simulink model "AnalizaSymulacyjna_z_opoznieniem"  (R2022b)
settings: Solver=VariableStepAuto  StartTime=0.0  StopTime=20  RelTol=1e-3
libraries: slpidlib x3
settings Model: Creator=hpiet  LastModifiedBy=hpiet

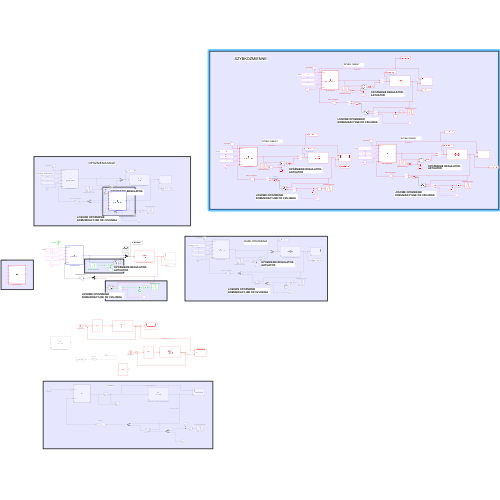
[thumbnail: Simulink's stored preview of the top-level diagram]
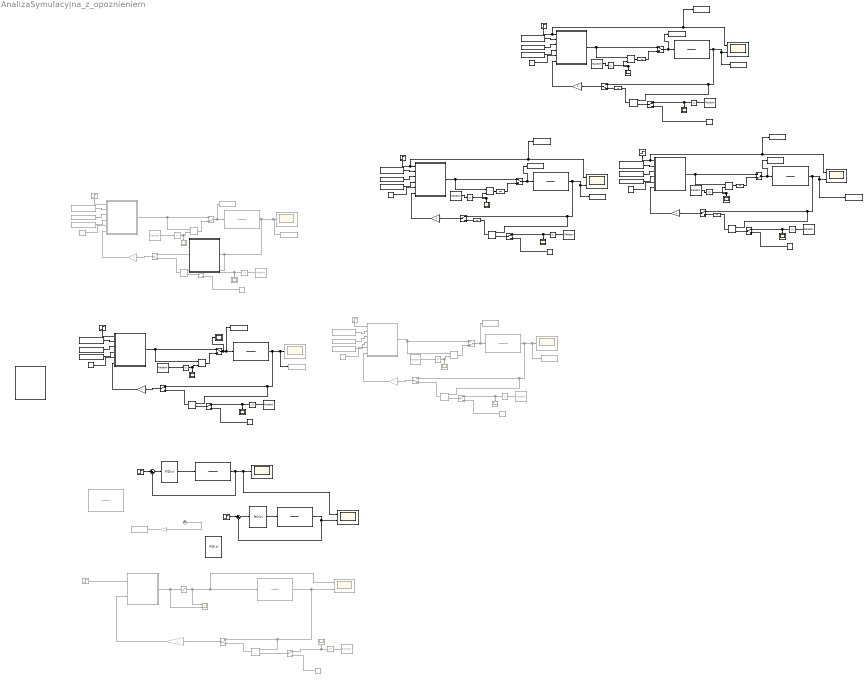
== system AnalizaSymulacyjna_z_opoznieniem ==
  note: SZYBKOZMIENNE
  note: SZYBKI OBIEKT
  note: OPOZNIENIA MALE
  note: WINDUP
  note: ORYGIAL
  note: DUZE OPOZNIENIA
  note: 23.33449541284404
  note: OPÓŹNIENIE REGULATOR-AKTUATOR
  note: LOSOWE OPÓŹNIENIE KOMUNIKACYJNE OD CZUJNIKA
  note: Z SATURACJA
  note: LOSOWE OPÓŹNIENIE KOMUNIKACYJNE OD CZUJNIKA
  note: OPÓŹNIENIE REGULATOR-AKTUATOR
  note: 23.33449541284404
  note: LOSOWE OPÓŹNIENIE KOMUNIKACYJNE OD CZUJNIKA
  note: OPÓŹNIENIE REGULATOR-AKTUATOR
  note: 23.33449541284404
  note: LOSOWE OPÓŹNIENIE KOMUNIKACYJNE OD CZUJNIKA
  note: 23.33449541284404
  note: OPÓŹNIENIE REGULATOR-AKTUATOR
  note: SZYBKI OBIEKT
  note: 23.33449541284404
  note: OPÓŹNIENIE REGULATOR-AKTUATOR
  note: LOSOWE OPÓŹNIENIE KOMUNIKACYJNE OD CZUJNIKA
  note: SZYBKI OBIEKT
  note: 23.33449541284404
  note: OPÓŹNIENIE REGULATOR-AKTUATOR
  note: LOSOWE OPÓŹNIENIE KOMUNIKACYJNE OD CZUJNIKA
  Abs{1,3,8..13} (8 alike) : Abs  SaturateOnIntegerOverflow=off
  Abs{2,4..7} (5 alike) : Abs  Commented=on  SaturateOnIntegerOverflow=off
  CZUJNIK1 : Gain  Commented=on
  Constant1 : Constant  Commented=on  Value=0.1
  Constant{6..7,10,12} (4 alike) : Constant  Value=0
  Constant{8..9,11,13} (4 alike) : Constant  Value=2
  Constant2 : Constant  Commented=on  Value=3.27
  Constant3 : Constant  Commented=on  Value=2
  Constant4 : Constant  Commented=on  Value=3.27
  Constant5 : Constant  Commented=on  Value=2
  Correction : Gain  Commented=on  Gain=0.1
  Discrete Transfer Fcn1 : DiscreteTransferFcn  Numerator=[0.001667]  Denominator=[1 -1]
  Discrete Transfer Fcn{5..8,10..11} (6 alike) : DiscreteTransferFcn  Denominator=[1]  SampleTime=0.02
  Discrete Transfer Fcn{2..4,9} (4 alike) : DiscreteTransferFcn  Numerator=[0.129]  Denominator=[1 -0.9355]  SampleTime=0.02
  "Example slow-changing plant " : TransferFcn  Commented=on  Numerator=[50]  Denominator=[300 1]
  IMITACJA CZUJNIKA{,3..5} (4 alike) : Gain
  IMITACJA CZUJNIKA1 : Gain  Commented=on
  IMITACJA CZUJNIKA2 : Gain  Commented=on
  KI : Constant  Value=1.2
  KI1 : Constant  Commented=on  Value=1.2
  KI2 : Constant  Commented=on  Value=1.2
  KI3 : Constant  Value=0.3
  KI4 : Constant  Value=0.3
  KI5 : Constant  Value=0.3
  KP : Constant  Value=23.3345
  KP1 : Constant  Commented=on  Value=23.33449541284404
  KP2 : Constant  Commented=on  Value=23.33449541284404
  KP3 : Constant  Value=0.08
  KP4 : Constant  Value=0.08
  KP5 : Constant  Value=0.08
  LOSOWE OPÓŹNIENIE1 : RandomNumber  Commented=on  Mean=0.1  Variance=0.0001  SampleTime=0.1
  MATLAB Function1 : MATLAB Function  Commented=on  TreatAsAtomicUnit=on
  Manual Switch{1,4,6..7,9} (5 alike) : ManualSwitch  Commented=on  CurrentSetting=0
  Manual Switch{3,10..16,19..20} (10 alike) : ManualSwitch
  Manual Switch17 : ManualSwitch  CurrentSetting=0
  Manual Switch18 : ManualSwitch  CurrentSetting=0
  Manual Switch2 : ManualSwitch  Commented=on
  Manual Switch5 : ManualSwitch  Commented=on
  Manual Switch8 : ManualSwitch  Commented=on
  PID CONTROLLER : MATLAB Function  TreatAsAtomicUnit=on
  PID CONTROLLER1 : MATLAB Function  Commented=on  TreatAsAtomicUnit=on  SystemSampleTime=0.5
  PID CONTROLLER2 : MATLAB Function  TreatAsAtomicUnit=on  SystemSampleTime=0.02
  PID CONTROLLER3 : MATLAB Function  TreatAsAtomicUnit=on  SystemSampleTime=0.5
  PID CONTROLLER4 : MATLAB Function  TreatAsAtomicUnit=on  SystemSampleTime=0.5
  PID CONTROLLER5 : MATLAB Function  Commented=on  TreatAsAtomicUnit=on  SystemSampleTime=0.5
  PID CONTROLLER6 : MATLAB Function  TreatAsAtomicUnit=on  SystemSampleTime=0.02
  PID CONTROLLER7 : MATLAB Function  TreatAsAtomicUnit=on  SystemSampleTime=0.02
  PID Controller : slpidlib/PID Controller  Controller=PID  Form=Parallel  TimeDomain=Discrete-time  UseExternalTs=off  SampleTime=-1  IntegratorMethod=Forward Euler  FilterMethod=Forward Euler  ControllerParametersSource=internal  P=16.762157558433  I=0.863667240387185  UseKiTs=off  D=11.7329946521911  N=1.01565558025853  UseFilter=on  TunerSelectOption=Transfer Function Based (PID Tuner App)  InitialConditionSource=internal  InitialConditionForIntegrator=0  InitialConditionForFilter=0  DifferentiatorICPrevScaledInput=0  ExternalReset=none  TrackingMode=off  Kt=1  LimitOutput=off  SatLimitsSource=internal  UpperSaturationLimit=inf  LowerSaturationLimit=-inf  LinearizeAsGain=on  AntiWindupMode=none  Kb=1  LimitIntegrator=off  UpperIntegratorSaturationLimit=inf  LowerIntegratorSaturationLimit=-inf  POutMin=[]  POutMax=[]  IOutMin=[]  IOutMax=[]  DOutMin=[]  DOutMax=[]  NOutMin=[]  NOutMax=[]  SumOutMin=[]  SumOutMax=[]  SaturationOutMin=[]  SaturationOutMax=[]  PParamMin=[]  PParamMax=[]  IParamMin=[]  IParamMax=[]  DParamMin=[]  DParamMax=[]  NParamMin=[]  NParamMax=[]  KbParamMin=[]  KbParamMax=[]  KtParamMin=[]  KtParamMax=[]  KbOutMin=[]  KbOutMax=[]  KtOutMin=[]  KtOutMax=[]  IntegratorOutMin=[]  IntegratorOutMax=[]  FilterOutMin=[]  FilterOutMax=[]  SumI1OutMin=[]  SumI1OutMax=[]  SumI2OutMin=[]  SumI2OutMax=[]  SumI3OutMin=[]  SumI3OutMax=[]  SumI4OutMin=[]  SumI4OutMax=[]  SumDOutMin=[]  SumDOutMax=[]  DifferentiatorOutMin=[]  DifferentiatorOutMax=[]  FilterDiffOutCoefMin=[]  FilterDiffOutCoefMax=[]  ReciprocalOutMin=[]  ReciprocalOutMax=[]  SumDenOutMin=[]  SumDenOutMax=[]  SumNumOutMin=[]  SumNumOutMax=[]  DivideOutMin=[]  DivideOutMax=[]  UdiffTsProdOutMin=[]  UdiffTsProdOutMax=[]  NTsProdOutMin=[]  NTsProdOutMax=[]  UintegralTsProdOutMin=[]  UintegralTsProdOutMax=[]  UngainTsProdOutMin=[]  UngainTsProdOutMax=[]  ClampingZeroOutDataTypeStr=Inherit: Inherit via back propagation  ClampingZeroOutMin=[]  ClampingZeroOutMax=[]  FilterDenConstantOutDataTypeStr=Inherit: Inherit via back propagation  FilterDenConstantOutMin=[]  FilterDenConstantOutMax=[]  PCopyOutDataTypeStr=Inherit: Inherit via back propagation  PCopyOutMin=[]  PCopyOutMax=[]  NCopyOutDataTypeStr=Inherit: Inherit via back propagation  NCopyOutMin=[]  NCopyOutMax=[]  IntegratorContinuousStateAttributes=''  IntegratorStateMustResolveToSignalObject=off  IntegratorRTWStateStorageClass=Auto  FilterContinuousStateAttributes=''  FilterStateMustResolveToSignalObject=off  FilterRTWStateStorageClass=Auto  ParallelPVariant=InternalParameters  IdealPVariant=Disabled  IVariant=InternalParameters  DVariant=InternalParameters  IntegratorVariant=Discrete  SatVariant=Disabled  AWVariant=Passthrough  PCopyVariant=Disabled  TRVariant=Disabled  FdbkBlocksVariant=Forward  IdealPFdbkVariant=Disabled  SatFdbkVariant=Disabled  DerivativeFilterVariant=ForwardEulerFilter  NVariant=InternalParameters  NCopyVariant=Disabled  FilterICVariant=InternalICsFilter  IntegratorICVariant=InternalICs  ExternalResetVariant=Disabled  TRSumVariant=Passthrough  SumFdbkVariant=Disabled  SumVariant=Sum_PID  TsampFilterVariant=InternalTs  TsampNgainVariant=Passthrough  TsampIntegralVariant=Passthrough  ExternalSaturationOutDataTypeStr=Inherit: Same as second input
  PID Controller1 : slpidlib/PID Controller  Controller=PID  Form=Parallel  TimeDomain=Discrete-time  UseExternalTs=off  SampleTime=-1  IntegratorMethod=Forward Euler  FilterMethod=Forward Euler  ControllerParametersSource=internal  P=16.762157558433  I=0.863667240387185  UseKiTs=off  D=11.7329946521911  N=1.01565558025853  UseFilter=on  TunerSelectOption=Transfer Function Based (PID Tuner App)  InitialConditionSource=internal  InitialConditionForIntegrator=0  InitialConditionForFilter=0  DifferentiatorICPrevScaledInput=0  ExternalReset=none  TrackingMode=off  Kt=1  LimitOutput=off  SatLimitsSource=internal  UpperSaturationLimit=inf  LowerSaturationLimit=-inf  LinearizeAsGain=on  AntiWindupMode=none  Kb=1  LimitIntegrator=off  UpperIntegratorSaturationLimit=inf  LowerIntegratorSaturationLimit=-inf  POutMin=[]  POutMax=[]  IOutMin=[]  IOutMax=[]  DOutMin=[]  DOutMax=[]  NOutMin=[]  NOutMax=[]  SumOutMin=[]  SumOutMax=[]  SaturationOutMin=[]  SaturationOutMax=[]  PParamMin=[]  PParamMax=[]  IParamMin=[]  IParamMax=[]  DParamMin=[]  DParamMax=[]  NParamMin=[]  NParamMax=[]  KbParamMin=[]  KbParamMax=[]  KtParamMin=[]  KtParamMax=[]  KbOutMin=[]  KbOutMax=[]  KtOutMin=[]  KtOutMax=[]  IntegratorOutMin=[]  IntegratorOutMax=[]  FilterOutMin=[]  FilterOutMax=[]  SumI1OutMin=[]  SumI1OutMax=[]  SumI2OutMin=[]  SumI2OutMax=[]  SumI3OutMin=[]  SumI3OutMax=[]  SumI4OutMin=[]  SumI4OutMax=[]  SumDOutMin=[]  SumDOutMax=[]  DifferentiatorOutMin=[]  DifferentiatorOutMax=[]  FilterDiffOutCoefMin=[]  FilterDiffOutCoefMax=[]  ReciprocalOutMin=[]  ReciprocalOutMax=[]  SumDenOutMin=[]  SumDenOutMax=[]  SumNumOutMin=[]  SumNumOutMax=[]  DivideOutMin=[]  DivideOutMax=[]  UdiffTsProdOutMin=[]  UdiffTsProdOutMax=[]  NTsProdOutMin=[]  NTsProdOutMax=[]  UintegralTsProdOutMin=[]  UintegralTsProdOutMax=[]  UngainTsProdOutMin=[]  UngainTsProdOutMax=[]  ClampingZeroOutDataTypeStr=Inherit: Inherit via back propagation  ClampingZeroOutMin=[]  ClampingZeroOutMax=[]  FilterDenConstantOutDataTypeStr=Inherit: Inherit via back propagation  FilterDenConstantOutMin=[]  FilterDenConstantOutMax=[]  PCopyOutDataTypeStr=Inherit: Inherit via back propagation  PCopyOutMin=[]  PCopyOutMax=[]  NCopyOutDataTypeStr=Inherit: Inherit via back propagation  NCopyOutMin=[]  NCopyOutMax=[]  IntegratorContinuousStateAttributes=''  IntegratorStateMustResolveToSignalObject=off  IntegratorRTWStateStorageClass=Auto  FilterContinuousStateAttributes=''  FilterStateMustResolveToSignalObject=off  FilterRTWStateStorageClass=Auto  ParallelPVariant=InternalParameters  IdealPVariant=Disabled  IVariant=InternalParameters  DVariant=InternalParameters  IntegratorVariant=Discrete  SatVariant=Disabled  AWVariant=Passthrough  PCopyVariant=Disabled  TRVariant=Disabled  FdbkBlocksVariant=Forward  IdealPFdbkVariant=Disabled  SatFdbkVariant=Disabled  DerivativeFilterVariant=ForwardEulerFilter  NVariant=InternalParameters  NCopyVariant=Disabled  FilterICVariant=InternalICsFilter  IntegratorICVariant=InternalICs  ExternalResetVariant=Disabled  TRSumVariant=Passthrough  SumFdbkVariant=Disabled  SumVariant=Sum_PID  TsampFilterVariant=InternalTs  TsampNgainVariant=Passthrough  TsampIntegralVariant=Passthrough  ExternalSaturationOutDataTypeStr=Inherit: Same as second input
  PID Controller2 : slpidlib/PID Controller  Controller=PID  Form=Parallel  TimeDomain=Discrete-time  UseExternalTs=off  SampleTime=0.02  IntegratorMethod=Forward Euler  FilterMethod=Forward Euler  ControllerParametersSource=internal  P=0.08  I=0.3  UseKiTs=off  D=0  N=0  UseFilter=on  TunerSelectOption=Transfer Function Based (PID Tuner App)  InitialConditionSource=internal  InitialConditionForIntegrator=0  InitialConditionForFilter=0  DifferentiatorICPrevScaledInput=0  ExternalReset=none  TrackingMode=off  Kt=1  LimitOutput=off  SatLimitsSource=internal  UpperSaturationLimit=inf  LowerSaturationLimit=-inf  LinearizeAsGain=on  AntiWindupMode=none  Kb=1  LimitIntegrator=off  UpperIntegratorSaturationLimit=inf  LowerIntegratorSaturationLimit=-inf  POutMin=[]  POutMax=[]  IOutMin=[]  IOutMax=[]  DOutMin=[]  DOutMax=[]  NOutMin=[]  NOutMax=[]  SumOutMin=[]  SumOutMax=[]  SaturationOutMin=[]  SaturationOutMax=[]  PParamMin=[]  PParamMax=[]  IParamMin=[]  IParamMax=[]  DParamMin=[]  DParamMax=[]  NParamMin=[]  NParamMax=[]  KbParamMin=[]  KbParamMax=[]  KtParamMin=[]  KtParamMax=[]  KbOutMin=[]  KbOutMax=[]  KtOutMin=[]  KtOutMax=[]  IntegratorOutMin=[]  IntegratorOutMax=[]  FilterOutMin=[]  FilterOutMax=[]  SumI1OutMin=[]  SumI1OutMax=[]  SumI2OutMin=[]  SumI2OutMax=[]  SumI3OutMin=[]  SumI3OutMax=[]  SumI4OutMin=[]  SumI4OutMax=[]  SumDOutMin=[]  SumDOutMax=[]  DifferentiatorOutMin=[]  DifferentiatorOutMax=[]  FilterDiffOutCoefMin=[]  FilterDiffOutCoefMax=[]  ReciprocalOutMin=[]  ReciprocalOutMax=[]  SumDenOutMin=[]  SumDenOutMax=[]  SumNumOutMin=[]  SumNumOutMax=[]  DivideOutMin=[]  DivideOutMax=[]  UdiffTsProdOutMin=[]  UdiffTsProdOutMax=[]  NTsProdOutMin=[]  NTsProdOutMax=[]  UintegralTsProdOutMin=[]  UintegralTsProdOutMax=[]  UngainTsProdOutMin=[]  UngainTsProdOutMax=[]  ClampingZeroOutDataTypeStr=Inherit: Inherit via back propagation  ClampingZeroOutMin=[]  ClampingZeroOutMax=[]  FilterDenConstantOutDataTypeStr=Inherit: Inherit via back propagation  FilterDenConstantOutMin=[]  FilterDenConstantOutMax=[]  PCopyOutDataTypeStr=Inherit: Inherit via back propagation  PCopyOutMin=[]  PCopyOutMax=[]  NCopyOutDataTypeStr=Inherit: Inherit via back propagation  NCopyOutMin=[]  NCopyOutMax=[]  IntegratorContinuousStateAttributes=''  IntegratorStateMustResolveToSignalObject=off  IntegratorRTWStateStorageClass=Auto  FilterContinuousStateAttributes=''  FilterStateMustResolveToSignalObject=off  FilterRTWStateStorageClass=Auto  ParallelPVariant=InternalParameters  IdealPVariant=Disabled  IVariant=InternalParameters  DVariant=InternalParameters  IntegratorVariant=Discrete  SatVariant=Disabled  AWVariant=Passthrough  PCopyVariant=Disabled  TRVariant=Disabled  FdbkBlocksVariant=Forward  IdealPFdbkVariant=Disabled  SatFdbkVariant=Disabled  DerivativeFilterVariant=ForwardEulerFilter  NVariant=InternalParameters  NCopyVariant=Disabled  FilterICVariant=InternalICsFilter  IntegratorICVariant=InternalICs  ExternalResetVariant=Disabled  TRSumVariant=Passthrough  SumFdbkVariant=Disabled  SumVariant=Sum_PID  TsampFilterVariant=InternalTs  TsampNgainVariant=Passthrough  TsampIntegralVariant=Passthrough  ExternalSaturationOutDataTypeStr=Inherit: Same as second input
  PRZYKŁADOWA TRANSMITANCJA : DiscreteTransferFcn  Numerator=[0.001667]  Denominator=[1 -1]
  PRZYKŁADOWA TRANSMITANCJA1 : DiscreteTransferFcn  Commented=on  Numerator=[0.001667]  Denominator=[1 -1]
  PRZYKŁADOWA TRANSMITANCJA2 : DiscreteTransferFcn  Commented=on  Numerator=[0.001667]  Denominator=[1 -1]
  PRZYKŁADOWY  OBIEKT WOLNOZMIENNY1 : TransferFcn  Commented=on  Numerator=[100]  Denominator=[300 1]
  RANDOM DELAY INIT : RandomNumber  Mean=1  Variance=0.0001  SampleTime=0.1
  RANDOM DELAY INIT1 : RandomNumber  Commented=on  Mean=0.1  Variance=0.0001  SampleTime=0.1
  RANDOM DELAY INIT{7,9..11} (4 alike) : RandomNumber  Mean=0.1  Variance=0.0001  SampleTime=0.02
  RANDOM DELAY INIT2 : RandomNumber  Mean=0.1  Variance=0.0001  SampleTime=0.1
  RANDOM DELAY INIT3 : RandomNumber  Commented=on  Mean=0.1  Variance=0.0001  SampleTime=0.1
  RANDOM DELAY INIT4 : RandomNumber  Commented=on  Mean=1  Variance=0.0001  SampleTime=0.1
  RANDOM DELAY INIT5 : RandomNumber  Commented=on  Mean=1  Variance=0.0001  SampleTime=0.1
  RANDOM DELAY INIT6 : RandomNumber  Mean=0.5  Variance=0.0001  SampleTime=0.02
  RANDOM DELAY INIT8 : RandomNumber  Mean=1  Variance=0.0001  SampleTime=0.02
  SET POINT : Step  Time=0  After=25  SampleTime=0.1
  SET POINT1 : Step  Commented=on  Time=0.5  After=25  SampleTime=0.1
  SET POINT2 : Step  Time=0
  SET POINT3 : Step  Time=0  SampleTime=0.02
  SET POINT4 : Step  Commented=on  Time=0  After=25  SampleTime=0.1
  SET POINT5 : Step  Commented=on  Time=0  After=25  SampleTime=0.1
  SET POINT6 : Step  Time=0  After=170  SampleTime=0.02
  SET POINT7 : Step  Time=0  After=170  SampleTime=0.02
  SET POINT8 : Step  Time=0  After=170  SampleTime=0.02
  Saturation1 : Saturate  Commented=on  UpperLimit=1200  LowerLimit=0
  Scope{,4,8..13} (8 alike) : Scope  Commented=on
  Scope{1..2,6,14..15,17..18,20..21,23} (10 alike) : Scope
  Scope{7,16,19,22} (4 alike) : Scope  NumInputPorts=2
  Scope3 : Scope  Commented=on  NumInputPorts=2
  Scope5 : Scope  Commented=on  NumInputPorts=2
  Sum : Sum  Inputs=|+-
  Sum1 : Sum  Commented=on  Inputs=+-|
  Sum2 : Sum  Inputs=|+-
  TS : Constant  Value=0.5  VectorParams1D=off
  TS1 : Constant  Commented=on  Value=0.5  VectorParams1D=off
  TS2 : Constant  Commented=on  Value=0.5  VectorParams1D=off
  TS3 : Constant  Value=0.02  VectorParams1D=off
  TS4 : Constant  Value=0.02  VectorParams1D=off
  TS5 : Constant  Value=0.02  VectorParams1D=off
  To Workspace : ToWorkspace  Commented=on  VariableName=simout  SaveFormat=Timeseries  SampleTime=-1
  To Workspace1 : ToWorkspace  Commented=on  VariableName=WYJSCIE  SaveFormat=Timeseries  SampleTime=-1
  To Workspace10 : ToWorkspace  VariableName=Sterujacy4  SaveFormat=Timeseries  SampleTime=-1
  To Workspace11 : ToWorkspace  VariableName=WYJSCIE5  SaveFormat=Timeseries  SampleTime=-1
  To Workspace12 : ToWorkspace  VariableName=Sterujacy5  SaveFormat=Timeseries  SampleTime=-1
  To Workspace13 : ToWorkspace  VariableName=Setpoint2  SaveFormat=Timeseries  SampleTime=-1
  To Workspace14 : ToWorkspace  VariableName=Setpoint1  SaveFormat=Timeseries  SampleTime=-1
  To Workspace15 : ToWorkspace  VariableName=Setpoint3  SaveFormat=Timeseries  SampleTime=-1
  To Workspace2 : ToWorkspace  Commented=on  VariableName=WYJSCIE1  SaveFormat=Timeseries  SampleTime=-1
  To Workspace3 : ToWorkspace  Commented=on  VariableName=WYJSCIE2  SaveFormat=Timeseries  SampleTime=-1
  To Workspace4 : ToWorkspace  VariableName=Sterujacy  SaveFormat=Timeseries  SampleTime=-1
  To Workspace5 : ToWorkspace  Commented=on  VariableName=Sterujacy1  SaveFormat=Timeseries  SampleTime=-1
  To Workspace6 : ToWorkspace  Commented=on  VariableName=Sterujacy2  SaveFormat=Timeseries  SampleTime=-1
  To Workspace7 : ToWorkspace  VariableName=WYJSCIE3  SaveFormat=Timeseries  SampleTime=-1
  To Workspace8 : ToWorkspace  VariableName=Sterujacy3  SaveFormat=Timeseries  SampleTime=-1
  To Workspace9 : ToWorkspace  VariableName=WYJSCIE4  SaveFormat=Timeseries  SampleTime=-1
  Variable Time Delay{1,3..4,6..7} (5 alike) : VariableTransportDelay  Commented=on  MaximumDelay=10
  Variable Time Delay{2,5,8..13} (8 alike) : VariableTransportDelay  MaximumDelay=10
  wires:
  Manual Switch16/1 -> Variable Time Delay5/2
  PRZYKŁADOWA TRANSMITANCJA/1 -> To Workspace1/1, Scope/1, Manual Switch13/1, Variable Time Delay5/1  "Y"
  Manual Switch13/1 -> IMITACJA CZUJNIKA/1
  Constant8/1 -> Manual Switch16/2
  RANDOM DELAY INIT/1 -> Abs1/1
  Variable Time Delay5/1 -> Manual Switch13/2
  Abs1/1 -> Manual Switch16/1, Scope1/1
  SET POINT/1 -> PID CONTROLLER3/1(SetPoint)
  IMITACJA CZUJNIKA/1 -> PID CONTROLLER3/6(Sensor)
  PID CONTROLLER3/1(u) -> Manual Switch3/1, Variable Time Delay2/1
  SET POINT1/1 -> MATLAB Function1/1(SetPoint)  "Sp"
  Variable Time Delay1/1 -> Manual Switch1/2
  LOSOWE OPÓŹNIENIE1/1 -> Abs2/1
  CZUJNIK1/1 -> MATLAB Function1/2(Sensor)
  Saturation1/1 -> Scope5/1, PRZYKŁADOWY  OBIEKT WOLNOZMIENNY1/1, Scope3/1  "SYGMAL STERUJĄCY"
  Abs2/1 -> Manual Switch2/1, Scope4/1
  MATLAB Function1/1(u) -> Saturation1/1, Scope5/2
  Constant1/1 -> Manual Switch2/2
  Manual Switch1/1 -> CZUJNIK1/1
  Manual Switch2/1 -> Variable Time Delay1/2
  PRZYKŁADOWY  OBIEKT WOLNOZMIENNY1/1 -> Manual Switch1/1, Variable Time Delay1/1, Scope3/2  "ODPOWIEDŹ UKŁADU"
  Sum/1 -> PID Controller/1
  SET POINT2/1 -> Sum/1
  PID Controller/1 -> Discrete Transfer Fcn1/1
  Discrete Transfer Fcn1/1 -> Scope7/1, Scope6/1, Sum/2  "AUTOREGULACJA"
  KI/1 -> PID CONTROLLER3/3(KI)
  Constant7/1 -> PID CONTROLLER3/4(KD)
  KP/1 -> PID CONTROLLER3/2(KP)
  TS/1 -> PID CONTROLLER3/5(TS)
  Correction/1 -> To Workspace/1
  Sum1/1 -> Correction/1
  RANDOM DELAY INIT2/1 -> Abs3/1
  Abs3/1 -> Scope2/1, Variable Time Delay2/2
  Variable Time Delay2/1 -> Manual Switch3/2
  Manual Switch3/1 -> Scope14/1, PRZYKŁADOWA TRANSMITANCJA/1, To Workspace4/1
  Discrete Transfer Fcn2/1 -> Scope7/2, Sum2/2  "BASIC PID"
  SET POINT3/1 -> Sum2/1
  Sum2/1 -> PID Controller2/1
  PID Controller2/1 -> Discrete Transfer Fcn2/1
  Variable Time Delay3/1 -> Manual Switch6/2
  KP1/1 -> PID CONTROLLER5/2(KP)
  TS1/1 -> PID CONTROLLER5/5(TS)
  RANDOM DELAY INIT3/1 -> Abs5/1
  KI1/1 -> PID CONTROLLER5/3(KI)
  Manual Switch6/1 -> PRZYKŁADOWA TRANSMITANCJA1/1, To Workspace5/1
  Abs4/1 -> Manual Switch5/1, Scope9/1
  Abs5/1 -> Scope10/1, Variable Time Delay3/2
  SET POINT4/1 -> PID CONTROLLER5/1(SetPoint)
  Constant2/1 -> PID CONTROLLER5/4(KD)
  Manual Switch5/1 -> Variable Time Delay4/2
  Variable Time Delay4/1 -> Manual Switch4/2
  RANDOM DELAY INIT1/1 -> Abs4/1
  PID CONTROLLER5/1(u) -> Manual Switch6/1, Variable Time Delay3/1
  Constant3/1 -> Manual Switch5/2
  Manual Switch4/1 -> IMITACJA CZUJNIKA1/1
  PRZYKŁADOWA TRANSMITANCJA1/1 -> To Workspace2/1, Scope8/1, Manual Switch4/1, Variable Time Delay4/1  "Y"
  IMITACJA CZUJNIKA1/1 -> PID CONTROLLER5/6(Sensor)
  Variable Time Delay6/1 -> Manual Switch9/2
  KP2/1 -> PID CONTROLLER1/2(KP)
  TS2/1 -> PID CONTROLLER1/5(TS)
  RANDOM DELAY INIT5/1 -> Abs7/1
  KI2/1 -> PID CONTROLLER1/3(KI)
  Manual Switch9/1 -> To Workspace6/1, PRZYKŁADOWA TRANSMITANCJA2/1
  Abs6/1 -> Manual Switch8/1, Scope12/1
  Abs7/1 -> Scope13/1, Variable Time Delay6/2
  SET POINT5/1 -> PID CONTROLLER1/1(SetPoint)
  Constant4/1 -> PID CONTROLLER1/4(KD)
  Manual Switch8/1 -> Variable Time Delay7/2
  Variable Time Delay7/1 -> Manual Switch7/2
  RANDOM DELAY INIT4/1 -> Abs6/1
  PID CONTROLLER1/1(u) -> Manual Switch9/1, Variable Time Delay6/1
  Constant5/1 -> Manual Switch8/2
  Manual Switch7/1 -> IMITACJA CZUJNIKA2/1
  PRZYKŁADOWA TRANSMITANCJA2/1 -> To Workspace3/1, Scope11/1, Manual Switch7/1, Variable Time Delay7/1  "Y"
  IMITACJA CZUJNIKA2/1 -> PID CONTROLLER1/6(Sensor)
  KP3/1 -> PID CONTROLLER2/2(KP)
  Variable Time Delay9/1 -> Discrete Transfer Fcn5/1
  TS3/1 -> PID CONTROLLER2/5(TS)
  Abs8/1 -> Manual Switch11/1, Scope17/1
  Abs9/1 -> Scope15/1, Variable Time Delay8/2
  KI3/1 -> PID CONTROLLER2/3(KI)
  Variable Time Delay8/1 -> Discrete Transfer Fcn6/1
  RANDOM DELAY INIT6/1 -> Abs8/1
  Manual Switch12/1 -> Discrete Transfer Fcn4/1, To Workspace8/1
  IMITACJA CZUJNIKA3/1 -> PID CONTROLLER2/6(Sensor)
  Discrete Transfer Fcn4/1 -> To Workspace7/1, Scope16/2, Manual Switch10/1, Variable Time Delay9/1  "Y"
  Manual Switch11/1 -> Variable Time Delay9/2
  Constant6/1 -> PID CONTROLLER2/4(KD)
  PID CONTROLLER2/1(u) -> Manual Switch12/1, Variable Time Delay8/1
  RANDOM DELAY INIT7/1 -> Abs9/1
  SET POINT6/1 -> To Workspace14/1, Scope16/1, PID CONTROLLER2/1(SetPoint)  "Wartość zadana"
  Constant9/1 -> Manual Switch11/2
  Manual Switch10/1 -> IMITACJA CZUJNIKA3/1
  Discrete Transfer Fcn5/1 -> Manual Switch10/2  "Y"
  Discrete Transfer Fcn6/1 -> Manual Switch12/2  "Y"
  SET POINT7/1 -> To Workspace15/1, Scope19/1, PID CONTROLLER6/1(SetPoint)  "Wartość zadana"
  Discrete Transfer Fcn8/1 -> Manual Switch17/2  "Y"
  RANDOM DELAY INIT9/1 -> Abs11/1
  Constant11/1 -> Manual Switch15/2
  Variable Time Delay10/1 -> Discrete Transfer Fcn8/1
  Abs11/1 -> Scope18/1, Variable Time Delay10/2
  IMITACJA CZUJNIKA4/1 -> PID CONTROLLER6/6(Sensor)
  RANDOM DELAY INIT8/1 -> Abs10/1
  Manual Switch17/1 -> Discrete Transfer Fcn3/1, To Workspace10/1
  Variable Time Delay11/1 -> Discrete Transfer Fcn7/1
  Abs10/1 -> Manual Switch15/1, Scope20/1
  Discrete Transfer Fcn3/1 -> To Workspace9/1, Scope19/2, Manual Switch14/1, Variable Time Delay11/1  "Y"
  KP4/1 -> PID CONTROLLER6/2(KP)
  PID CONTROLLER6/1(u) -> Manual Switch17/1, Variable Time Delay10/1
  Constant10/1 -> PID CONTROLLER6/4(KD)
  TS4/1 -> PID CONTROLLER6/5(TS)
  Manual Switch15/1 -> Variable Time Delay11/2
  Manual Switch14/1 -> IMITACJA CZUJNIKA4/1
  Discrete Transfer Fcn7/1 -> Manual Switch14/2  "Y"
  KI4/1 -> PID CONTROLLER6/3(KI)
  SET POINT8/1 -> To Workspace13/1, Scope22/1, PID CONTROLLER7/1(SetPoint)  "Wartość zadana"
  Discrete Transfer Fcn11/1 -> Manual Switch20/2  "Y"
  RANDOM DELAY INIT11/1 -> Abs13/1
  Constant13/1 -> Manual Switch19/2
  Variable Time Delay12/1 -> Discrete Transfer Fcn11/1
  Abs13/1 -> Scope21/1, Variable Time Delay12/2
  IMITACJA CZUJNIKA5/1 -> PID CONTROLLER7/6(Sensor)
  RANDOM DELAY INIT10/1 -> Abs12/1
  Manual Switch20/1 -> Discrete Transfer Fcn9/1, To Workspace12/1
  Variable Time Delay13/1 -> Discrete Transfer Fcn10/1
  Abs12/1 -> Manual Switch19/1, Scope23/1
  Discrete Transfer Fcn9/1 -> To Workspace11/1, Scope22/2, Manual Switch18/1, Variable Time Delay13/1  "Y"
  KP5/1 -> PID CONTROLLER7/2(KP)
  PID CONTROLLER7/1(u) -> Manual Switch20/1, Variable Time Delay12/1
  Constant12/1 -> PID CONTROLLER7/4(KD)
  TS5/1 -> PID CONTROLLER7/5(TS)
  Manual Switch19/1 -> Variable Time Delay13/2
  Manual Switch18/1 -> IMITACJA CZUJNIKA5/1
  Discrete Transfer Fcn10/1 -> Manual Switch18/2  "Y"
  KI5/1 -> PID CONTROLLER7/3(KI)

== matlab function AnalizaSymulacyjna_z_opoznieniem/PID CONTROLLER6 ==
  settings: updateMethod=DISCRETE
  data: SetPoint input; KP input; KI input; KD input; TS input; u output; Sensor input
function u = PID_CONTROLLER(SetPoint, KP, KI, KD, TS, Sensor) 

persistent init u1 u2 e1 e2 KU1 KU2 KE0 KE1 KE2 integral_error  sat_upper sat_lower tmp ;

if isempty(init)
%INICJALIZACJA FUNKCJI Z SKRYPTU MATLAB
[KU1,KU2,KE0,KE1,KE2]=PID_init(KP,KI,KD,TS);
e2=0;
e1=0;
u2=0;
u1=0;
sat_upper = 100;
sat_lower= 0;
integral_error=0;
KW=0.1;
tmp=KW*(-KU1- KU2)/2;
init=1;
end

%Definicja uchybu i równanie sterowania PID
e0=SetPoint-Sensor;

u0 = -KU1*u1 - KU2 * u2 + (KE0*e0) + (KE1*e1) + (KE2*e2)+tmp*integral_error;
if(u0 > sat_upper) 
    integral_error=  sat_upper-u0;
elseif ( u0 < sat_lower)
    integral_error= sat_lower-u0;
else
    integral_error=0;
end
e2=e1;
e1=e0;
u2=u1;
u1=u0;

if(u0 > sat_upper) 
    u0= sat_upper;
elseif ( u0 < sat_lower)
    u0= sat_lower;    
end


u=u0;
end





%BZDURY
% integral_error=integral_error + KE0*e0;
% presat_integral_error = integral_error;
% PD=(KE1*e1) + (KE2*e2);
% 
% u0 = -(KU1*u1) - (KU2 * u2) + (KE0*e0) + (KE1*e1) + (KE2*e2);
% 
% %ANTY WINDUP
% 
% if(u0 > sat_upper)
%     u0= sat_upper;
% elseif ( u0 < sat_lower)
%     u0= sat_lower;
% end
% 
% 
% integral_error = presat_integral_error + (u0 - (PD))/(KE0);
% 
% e2=e1;
% e1=e0;
% u2=u1;
% u1=u0;
% 
% u=u0;
% 
% end

== matlab function AnalizaSymulacyjna_z_opoznieniem/PID CONTROLLER7 ==
  settings: updateMethod=DISCRETE
  data: SetPoint input; KP input; KI input; KD input; TS input; u output; Sensor input
function u = PID_CONTROLLER(SetPoint, KP, KI, KD, TS, Sensor) 

persistent init u1 u2 e1 e2 KU1 KU2 KE0 KE1 KE2 integral_error  sat_upper sat_lower tmp ;

if isempty(init)
%INICJALIZACJA FUNKCJI Z SKRYPTU MATLAB
[KU1,KU2,KE0,KE1,KE2]=PID_init(KP,KI,KD,TS);
e2=0;
e1=0;
u2=0;
u1=0;
sat_upper = 100;
sat_lower= 0;
integral_error=0;
KW=0.1;
tmp=KW*(-KU1- KU2)/2;
init=1;
end

%Definicja uchybu i równanie sterowania PID
e0=SetPoint-Sensor;

u0 = -KU1*u1 - KU2 * u2 + (KE0*e0) + (KE1*e1) + (KE2*e2)+tmp*integral_error;
if(u0 > sat_upper) 
    integral_error=  sat_upper-u0;
elseif ( u0 < sat_lower)
    integral_error= sat_lower-u0;
else
    integral_error=0;
end
e2=e1;
e1=e0;
u2=u1;
u1=u0;

if(u0 > sat_upper) 
    u0= sat_upper;
elseif ( u0 < sat_lower)
    u0= sat_lower;    
end


u=u0;
end





%BZDURY
% integral_error=integral_error + KE0*e0;
% presat_integral_error = integral_error;
% PD=(KE1*e1) + (KE2*e2);
% 
% u0 = -(KU1*u1) - (KU2 * u2) + (KE0*e0) + (KE1*e1) + (KE2*e2);
% 
% %ANTY WINDUP
% 
% if(u0 > sat_upper)
%     u0= sat_upper;
% elseif ( u0 < sat_lower)
%     u0= sat_lower;
% end
% 
% 
% integral_error = presat_integral_error + (u0 - (PD))/(KE0);
% 
% e2=e1;
% e1=e0;
% u2=u1;
% u1=u0;
% 
% u=u0;
% 
% end

== matlab function AnalizaSymulacyjna_z_opoznieniem/MATLAB Function1 ==
  settings: updateMethod=DISCRETE
  data: SetPoint input; u output; Sensor input
function u = fcn(SetPoint,Sensor) 
persistent init e2 e1 u2 u1 ku1 ku2 ke0 ke1 ke2 ;

if isempty(init) %wykonuje się tylko raz
Kp = 0.0975043176181261;
Ki =0.00404938736460088;
Kd = 0.148625801524361;
FCoef = 0.191342781331139;
Ts=0.01; %czas próbki

%e0=Sp


e2=0;
e1=0;
u2=0;
u1=0;

a0 = (1 + FCoef * Ts);
a1 = -(2 + FCoef * Ts);
a2 = 1;

b0=Kp*(1+FCoef * Ts) + Ki*Ts*(1+ FCoef*Ts) + Kd*FCoef;
b1= -(Kp*(2+FCoef*Ts) + Ki*Ts + 2*Kd*FCoef);
b2=Kp + Kd * FCoef;

%uproszczenie równania
ku1=a1/a0;
ku2=a2/a0;
ke0=b0/a0;
ke1=b1/a0;
ke2=b2/a0;
init=1;
end

e0=SetPoint-Sensor;
u0 = -(ku1*u1) - (ku2 * u2) + (ke0*e0) + (ke1*e1) + (ke2*e2);

e2=e1;
e1=e0;
u2=u1;
u1=u0;

u=u0;
end

== matlab function AnalizaSymulacyjna_z_opoznieniem/PID CONTROLLER1 ==
  settings: updateMethod=DISCRETE
  data: SetPoint input; KP input; KI input; KD input; TS input; u output; Sensor input
function u = PID_CONTROLLER(SetPoint, KP, KI, KD, TS, Sensor) 

persistent init u1 u2 e1 e2 KU1 KU2 KE0 KE1 KE2 integral_error  sat_upper sat_lower tmp ;

if isempty(init)
%INICJALIZACJA FUNKCJI Z SKRYPTU MATLAB
[KU1,KU2,KE0,KE1,KE2]=PID_init(KP,KI,KD,TS);
e2=0;
e1=0;
u2=0;
u1=0;
sat_upper = 100;
sat_lower= 0;
integral_error=0;
KW=0.1;
tmp=KW*(-KU1- KU2)/2;
init=1;
end

%Definicja uchybu i równanie sterowania PID
e0=SetPoint-Sensor;

u0 = -KU1*u1 - KU2 * u2 + (KE0*e0) + (KE1*e1) + (KE2*e2)+tmp*integral_error;
if(u0 > sat_upper) 
    integral_error=  sat_upper-u0;
elseif ( u0 < sat_lower)
    integral_error= sat_lower-u0;
else
    integral_error=0;
end
e2=e1;
e1=e0;
u2=u1;
u1=u0;

if(u0 > sat_upper) 
    u0= sat_upper;
elseif ( u0 < sat_lower)
    u0= sat_lower;    
end


u=u0;
end





%BZDURY
% integral_error=integral_error + KE0*e0;
% presat_integral_error = integral_error;
% PD=(KE1*e1) + (KE2*e2);
% 
% u0 = -(KU1*u1) - (KU2 * u2) + (KE0*e0) + (KE1*e1) + (KE2*e2);
% 
% %ANTY WINDUP
% 
% if(u0 > sat_upper)
%     u0= sat_upper;
% elseif ( u0 < sat_lower)
%     u0= sat_lower;
% end
% 
% 
% integral_error = presat_integral_error + (u0 - (PD))/(KE0);
% 
% e2=e1;
% e1=e0;
% u2=u1;
% u1=u0;
% 
% u=u0;
% 
% end

== matlab function AnalizaSymulacyjna_z_opoznieniem/PID CONTROLLER2 ==
  settings: updateMethod=DISCRETE
  data: SetPoint input; KP input; KI input; KD input; TS input; u output; Sensor input
function u = PID_CONTROLLER(SetPoint, KP, KI, KD, TS, Sensor) 

persistent init u1 u2 e1 e2 KU1 KU2 KE0 KE1 KE2 integral_error  sat_upper sat_lower tmp ;

if isempty(init)
%INICJALIZACJA FUNKCJI Z SKRYPTU MATLAB
[KU1,KU2,KE0,KE1,KE2]=PID_init(KP,KI,KD,TS);
e2=0;
e1=0;
u2=0;
u1=0;
sat_upper = 100;
sat_lower= 0;
integral_error=0;
KW=0.1;
tmp=KW*(-KU1- KU2)/2;
init=1;
end

%Definicja uchybu i równanie sterowania PID
e0=SetPoint-Sensor;

u0 = -KU1*u1 - KU2 * u2 + (KE0*e0) + (KE1*e1) + (KE2*e2)+tmp*integral_error;
if(u0 > sat_upper) 
    integral_error=  sat_upper-u0;
elseif ( u0 < sat_lower)
    integral_error= sat_lower-u0;
else
    integral_error=0;
end
e2=e1;
e1=e0;
u2=u1;
u1=u0;

if(u0 > sat_upper) 
    u0= sat_upper;
elseif ( u0 < sat_lower)
    u0= sat_lower;    
end


u=u0;
end





%BZDURY
% integral_error=integral_error + KE0*e0;
% presat_integral_error = integral_error;
% PD=(KE1*e1) + (KE2*e2);
% 
% u0 = -(KU1*u1) - (KU2 * u2) + (KE0*e0) + (KE1*e1) + (KE2*e2);
% 
% %ANTY WINDUP
% 
% if(u0 > sat_upper)
%     u0= sat_upper;
% elseif ( u0 < sat_lower)
%     u0= sat_lower;
% end
% 
% 
% integral_error = presat_integral_error + (u0 - (PD))/(KE0);
% 
% e2=e1;
% e1=e0;
% u2=u1;
% u1=u0;
% 
% u=u0;
% 
% end

== matlab function AnalizaSymulacyjna_z_opoznieniem/PID CONTROLLER ==
  settings: updateMethod=DISCRETE
  data: SetPoint input; KP input; KI input; KD input; TS input; u output; Sensor input
function u = PID_CONTROLLER(SetPoint, KP, KI, KD, TS, Sensor) 

persistent init u1 u2 e1 e2 KU1 KU2 KE0 KE1 KE2 integral_error sat_upper sat_lower Kfi Korektor;

if isempty(init)
%INICJALIZACJA FUNKCJI Z SKRYPTU MATLAB
[KU1,KU2,KE0,KE1,KE2]=PID_init(KP,KI,KD,TS);
e2=0;
e1=0;
u2=0;
u1=0;
sat_upper = 100;
sat_lower= 0;
Kfi=0.1; %korekcja saturacji
integral_error=0;
Korektor=Kfi*(-KU1-KU2)/2;
init=1;

end

%Definicja uchybu i równanie sterowania PID
e0=SetPoint-Sensor;
u0 = -(KU1*u1) - (KU2 * u2) + (KE0*e0) + (KE1*e1) + (KE2*e2) + Korektor*integral_error;


if(u0 > sat_upper)
    integral_error =sat_upper-u0;
elseif ( u0 < sat_lower)
    integral_error = sat_lower-u0;
else
    integral_error=0;
end

e2=e1;
e1=e0;
u2=u1;
u1=u0;


if(u0 > sat_upper)
    u0= sat_upper;
elseif ( u0 < sat_lower)
    u0= sat_lower;
end


u=u0;
end

== matlab function AnalizaSymulacyjna_z_opoznieniem/PID CONTROLLER3 ==
  settings: updateMethod=DISCRETE
  data: SetPoint input; KP input; KI input; KD input; TS input; u output; Sensor input
function u = PID_CONTROLLER(SetPoint, KP, KI, KD, TS, Sensor) 

persistent init u1 u2 e1 e2 KU1 KU2 KE0 KE1 KE2 integral_error  sat_upper sat_lower tmp ;

if isempty(init)
%INICJALIZACJA FUNKCJI Z SKRYPTU MATLAB
[KU1,KU2,KE0,KE1,KE2]=PID_init(KP,KI,KD,TS);
e2=0;
e1=0;
u2=0;
u1=0;
sat_upper = 100;
sat_lower= 0;
integral_error=0;
KW=0.1;
tmp=KW*(-KU1- KU2)/2;
init=1;
end

%Definicja uchybu i równanie sterowania PID
e0=SetPoint-Sensor;

u0 = -KU1*u1 - KU2 * u2 + (KE0*e0) + (KE1*e1) + (KE2*e2)+tmp*integral_error;
if(u0 > sat_upper) 
    integral_error=  sat_upper-u0;
elseif ( u0 < sat_lower)
    integral_error= sat_lower-u0;
else
    integral_error=0;
end
e2=e1;
e1=e0;
u2=u1;
u1=u0;

if(u0 > sat_upper) 
    u0= sat_upper;
elseif ( u0 < sat_lower)
    u0= sat_lower;    
end


u=u0;
end





%BZDURY
% integral_error=integral_error + KE0*e0;
% presat_integral_error = integral_error;
% PD=(KE1*e1) + (KE2*e2);
% 
% u0 = -(KU1*u1) - (KU2 * u2) + (KE0*e0) + (KE1*e1) + (KE2*e2);
% 
% %ANTY WINDUP
% 
% if(u0 > sat_upper)
%     u0= sat_upper;
% elseif ( u0 < sat_lower)
%     u0= sat_lower;
% end
% 
% 
% integral_error = presat_integral_error + (u0 - (PD))/(KE0);
% 
% e2=e1;
% e1=e0;
% u2=u1;
% u1=u0;
% 
% u=u0;
% 
% end

== matlab function AnalizaSymulacyjna_z_opoznieniem/PID CONTROLLER4 ==
  settings: updateMethod=DISCRETE
  data: SetPoint input; KP input; KI input; KD input; TS input; u output; Sensor input
function u = PID_CONTROLLER(SetPoint, KP, KI, KD, TS, Sensor) 

persistent init u1 u2 e1 e2 KU1 KU2 KE0 KE1 KE2 integral_error  sat_upper sat_lower tmp ;

if isempty(init)
%INICJALIZACJA FUNKCJI Z SKRYPTU MATLAB
[KU1,KU2,KE0,KE1,KE2]=PID_init(KP,KI,KD,TS);
e2=0;
e1=0;
u2=0;
u1=0;
sat_upper = 100;
sat_lower= 0;
integral_error=0;
KW=0.1;
tmp=KW*(-KU1- KU2)/2;
init=1;
end

%Definicja uchybu i równanie sterowania PID
e0=SetPoint-Sensor;

u0 = -KU1*u1 - KU2 * u2 + (KE0*e0) + (KE1*e1) + (KE2*e2)+tmp*integral_error;
if(u0 > sat_upper) 
    integral_error=  sat_upper-u0;
elseif ( u0 < sat_lower)
    integral_error= sat_lower-u0;
else
    integral_error=0;
end
e2=e1;
e1=e0;
u2=u1;
u1=u0;

if(u0 > sat_upper) 
    u0= sat_upper;
elseif ( u0 < sat_lower)
    u0= sat_lower;    
end


u=u0;
end





%BZDURY
% integral_error=integral_error + KE0*e0;
% presat_integral_error = integral_error;
% PD=(KE1*e1) + (KE2*e2);
% 
% u0 = -(KU1*u1) - (KU2 * u2) + (KE0*e0) + (KE1*e1) + (KE2*e2);
% 
% %ANTY WINDUP
% 
% if(u0 > sat_upper)
%     u0= sat_upper;
% elseif ( u0 < sat_lower)
%     u0= sat_lower;
% end
% 
% 
% integral_error = presat_integral_error + (u0 - (PD))/(KE0);
% 
% e2=e1;
% e1=e0;
% u2=u1;
% u1=u0;
% 
% u=u0;
% 
% end

== matlab function AnalizaSymulacyjna_z_opoznieniem/PID CONTROLLER5 ==
  settings: updateMethod=DISCRETE
  data: SetPoint input; KP input; KI input; KD input; TS input; u output; Sensor input
function u = PID_CONTROLLER(SetPoint, KP, KI, KD, TS, Sensor) 

persistent init u1 u2 e1 e2 KU1 KU2 KE0 KE1 KE2 integral_error  sat_upper sat_lower tmp ;

if isempty(init)
%INICJALIZACJA FUNKCJI Z SKRYPTU MATLAB
[KU1,KU2,KE0,KE1,KE2]=PID_init(KP,KI,KD,TS);
e2=0;
e1=0;
u2=0;
u1=0;
sat_upper = 100;
sat_lower= 0;
integral_error=0;
KW=0.1;
tmp=KW*(-KU1- KU2)/2;
init=1;
end

%Definicja uchybu i równanie sterowania PID
e0=SetPoint-Sensor;

u0 = -KU1*u1 - KU2 * u2 + (KE0*e0) + (KE1*e1) + (KE2*e2)+tmp*integral_error;
if(u0 > sat_upper) 
    integral_error=  sat_upper-u0;
elseif ( u0 < sat_lower)
    integral_error= sat_lower-u0;
else
    integral_error=0;
end
e2=e1;
e1=e0;
u2=u1;
u1=u0;

if(u0 > sat_upper) 
    u0= sat_upper;
elseif ( u0 < sat_lower)
    u0= sat_lower;    
end


u=u0;
end





%BZDURY
% integral_error=integral_error + KE0*e0;
% presat_integral_error = integral_error;
% PD=(KE1*e1) + (KE2*e2);
% 
% u0 = -(KU1*u1) - (KU2 * u2) + (KE0*e0) + (KE1*e1) + (KE2*e2);
% 
% %ANTY WINDUP
% 
% if(u0 > sat_upper)
%     u0= sat_upper;
% elseif ( u0 < sat_lower)
%     u0= sat_lower;
% end
% 
% 
% integral_error = presat_integral_error + (u0 - (PD))/(KE0);
% 
% e2=e1;
% e1=e0;
% u2=u1;
% u1=u0;
% 
% u=u0;
% 
% end
